simulink model "waterTankBurner"  (R2014b)
settings: Solver=ode1  StartTime=0.0  StopTime=100  FixedStep=0.0001  MaxStep=0.0001  RelTol=1e-3
(part 4 of 4)

== matlab function waterTankBurner/waterTank38/MATLAB Function1 ==
  data: x input; ode1 output; ode2 output; ode3 output; ode4 output
function [ode1,ode2,ode3,ode4] = ODEs(x)
%#codegen
K=0.075;
h=150;
ode1=0;
ode2=K*(h-x);
ode3=0;
ode4=-K*x;

== matlab function waterTankBurner/waterTank39/MATLAB Function ==
  data: q input; ON input; OFF input; x input; qNext output; reset output


function [qNext,reset]  = phi(q,  ON, OFF,x)
%#codegen


if q==1 % q=1, tank is in t1
    if ON==0
        qNext=1;
        reset=0;
    elseif ON==1
        qNext=2;
        reset=1;
    else
        qNext=-1;
        reset=-1;
    end;
    
elseif q==2 % q=2, tank is in t2
    if x<100 && OFF==0
        qNext=2;
        reset=0;
    elseif x>=100
        qNext=3;
        reset=1;
    elseif x<100 && OFF==1
        qNext=4;
        reset=1;
    else
        qNext=-1;
        reset=-1;
    end;

elseif q==3 % q=3, tank is in state t3
    if OFF==0
        qNext=3;
        reset=0;
    elseif OFF==1
        qNext=4;
        reset=1;
    else
        qNext=-1;
        reset=-1;
    end;
elseif q==4 % q=4, tank is in state t4
    if x>20 && ON==0
        qNext=4;
        reset=0;
    elseif x<=20
        qNext=1;
        reset=1;
    elseif x>20 && ON==1
        qNext=2;
        reset=1;
    else
        qNext=-1;
        reset=-1;
    end;
else
    qNext=-1; %this should never execute
    reset=-1;%this should never execute
end

== matlab function waterTankBurner/waterTank39/MATLAB Function1 ==
  data: x input; ode1 output; ode2 output; ode3 output; ode4 output
function [ode1,ode2,ode3,ode4] = ODEs(x)
%#codegen
K=0.075;
h=150;
ode1=0;
ode2=K*(h-x);
ode3=0;
ode4=-K*x;

== matlab function waterTankBurner/waterTank40/MATLAB Function ==
  data: q input; ON input; OFF input; x input; qNext output; reset output


function [qNext,reset]  = phi(q,  ON, OFF,x)
%#codegen


if q==1 % q=1, tank is in t1
    if ON==0
        qNext=1;
        reset=0;
    elseif ON==1
        qNext=2;
        reset=1;
    else
        qNext=-1;
        reset=-1;
    end;
    
elseif q==2 % q=2, tank is in t2
    if x<100 && OFF==0
        qNext=2;
        reset=0;
    elseif x>=100
        qNext=3;
        reset=1;
    elseif x<100 && OFF==1
        qNext=4;
        reset=1;
    else
        qNext=-1;
        reset=-1;
    end;

elseif q==3 % q=3, tank is in state t3
    if OFF==0
        qNext=3;
        reset=0;
    elseif OFF==1
        qNext=4;
        reset=1;
    else
        qNext=-1;
        reset=-1;
    end;
elseif q==4 % q=4, tank is in state t4
    if x>20 && ON==0
        qNext=4;
        reset=0;
    elseif x<=20
        qNext=1;
        reset=1;
    elseif x>20 && ON==1
        qNext=2;
        reset=1;
    else
        qNext=-1;
        reset=-1;
    end;
else
    qNext=-1; %this should never execute
    reset=-1;%this should never execute
end

== matlab function waterTankBurner/waterTank40/MATLAB Function1 ==
  data: x input; ode1 output; ode2 output; ode3 output; ode4 output
function [ode1,ode2,ode3,ode4] = ODEs(x)
%#codegen
K=0.075;
h=150;
ode1=0;
ode2=K*(h-x);
ode3=0;
ode4=-K*x;

== matlab function waterTankBurner/waterTank41/MATLAB Function ==
  data: q input; ON input; OFF input; x input; qNext output; reset output


function [qNext,reset]  = phi(q,  ON, OFF,x)
%#codegen


if q==1 % q=1, tank is in t1
    if ON==0
        qNext=1;
        reset=0;
    elseif ON==1
        qNext=2;
        reset=1;
    else
        qNext=-1;
        reset=-1;
    end;
    
elseif q==2 % q=2, tank is in t2
    if x<100 && OFF==0
        qNext=2;
        reset=0;
    elseif x>=100
        qNext=3;
        reset=1;
    elseif x<100 && OFF==1
        qNext=4;
        reset=1;
    else
        qNext=-1;
        reset=-1;
    end;

elseif q==3 % q=3, tank is in state t3
    if OFF==0
        qNext=3;
        reset=0;
    elseif OFF==1
        qNext=4;
        reset=1;
    else
        qNext=-1;
        reset=-1;
    end;
elseif q==4 % q=4, tank is in state t4
    if x>20 && ON==0
        qNext=4;
        reset=0;
    elseif x<=20
        qNext=1;
        reset=1;
    elseif x>20 && ON==1
        qNext=2;
        reset=1;
    else
        qNext=-1;
        reset=-1;
    end;
else
    qNext=-1; %this should never execute
    reset=-1;%this should never execute
end

== matlab function waterTankBurner/waterTank41/MATLAB Function1 ==
  data: x input; ode1 output; ode2 output; ode3 output; ode4 output
function [ode1,ode2,ode3,ode4] = ODEs(x)
%#codegen
K=0.075;
h=150;
ode1=0;
ode2=K*(h-x);
ode3=0;
ode4=-K*x;

== matlab function waterTankBurner/waterTank42/MATLAB Function ==
  data: q input; ON input; OFF input; x input; qNext output; reset output


function [qNext,reset]  = phi(q,  ON, OFF,x)
%#codegen


if q==1 % q=1, tank is in t1
    if ON==0
        qNext=1;
        reset=0;
    elseif ON==1
        qNext=2;
        reset=1;
    else
        qNext=-1;
        reset=-1;
    end;
    
elseif q==2 % q=2, tank is in t2
    if x<100 && OFF==0
        qNext=2;
        reset=0;
    elseif x>=100
        qNext=3;
        reset=1;
    elseif x<100 && OFF==1
        qNext=4;
        reset=1;
    else
        qNext=-1;
        reset=-1;
    end;

elseif q==3 % q=3, tank is in state t3
    if OFF==0
        qNext=3;
        reset=0;
    elseif OFF==1
        qNext=4;
        reset=1;
    else
        qNext=-1;
        reset=-1;
    end;
elseif q==4 % q=4, tank is in state t4
    if x>20 && ON==0
        qNext=4;
        reset=0;
    elseif x<=20
        qNext=1;
        reset=1;
    elseif x>20 && ON==1
        qNext=2;
        reset=1;
    else
        qNext=-1;
        reset=-1;
    end;
else
    qNext=-1; %this should never execute
    reset=-1;%this should never execute
end

== matlab function waterTankBurner/waterTank42/MATLAB Function1 ==
  data: x input; ode1 output; ode2 output; ode3 output; ode4 output
function [ode1,ode2,ode3,ode4] = ODEs(x)
%#codegen
K=0.075;
h=150;
ode1=0;
ode2=K*(h-x);
ode3=0;
ode4=-K*x;

== matlab function waterTankBurner/waterTank43/MATLAB Function ==
  data: q input; ON input; OFF input; x input; qNext output; reset output


function [qNext,reset]  = phi(q,  ON, OFF,x)
%#codegen


if q==1 % q=1, tank is in t1
    if ON==0
        qNext=1;
        reset=0;
    elseif ON==1
        qNext=2;
        reset=1;
    else
        qNext=-1;
        reset=-1;
    end;
    
elseif q==2 % q=2, tank is in t2
    if x<100 && OFF==0
        qNext=2;
        reset=0;
    elseif x>=100
        qNext=3;
        reset=1;
    elseif x<100 && OFF==1
        qNext=4;
        reset=1;
    else
        qNext=-1;
        reset=-1;
    end;

elseif q==3 % q=3, tank is in state t3
    if OFF==0
        qNext=3;
        reset=0;
    elseif OFF==1
        qNext=4;
        reset=1;
    else
        qNext=-1;
        reset=-1;
    end;
elseif q==4 % q=4, tank is in state t4
    if x>20 && ON==0
        qNext=4;
        reset=0;
    elseif x<=20
        qNext=1;
        reset=1;
    elseif x>20 && ON==1
        qNext=2;
        reset=1;
    else
        qNext=-1;
        reset=-1;
    end;
else
    qNext=-1; %this should never execute
    reset=-1;%this should never execute
end

== matlab function waterTankBurner/waterTank43/MATLAB Function1 ==
  data: x input; ode1 output; ode2 output; ode3 output; ode4 output
function [ode1,ode2,ode3,ode4] = ODEs(x)
%#codegen
K=0.075;
h=150;
ode1=0;
ode2=K*(h-x);
ode3=0;
ode4=-K*x;

== matlab function waterTankBurner/waterTank44/MATLAB Function ==
  data: q input; ON input; OFF input; x input; qNext output; reset output


function [qNext,reset]  = phi(q,  ON, OFF,x)
%#codegen


if q==1 % q=1, tank is in t1
    if ON==0
        qNext=1;
        reset=0;
    elseif ON==1
        qNext=2;
        reset=1;
    else
        qNext=-1;
        reset=-1;
    end;
    
elseif q==2 % q=2, tank is in t2
    if x<100 && OFF==0
        qNext=2;
        reset=0;
    elseif x>=100
        qNext=3;
        reset=1;
    elseif x<100 && OFF==1
        qNext=4;
        reset=1;
    else
        qNext=-1;
        reset=-1;
    end;

elseif q==3 % q=3, tank is in state t3
    if OFF==0
        qNext=3;
        reset=0;
    elseif OFF==1
        qNext=4;
        reset=1;
    else
        qNext=-1;
        reset=-1;
    end;
elseif q==4 % q=4, tank is in state t4
    if x>20 && ON==0
        qNext=4;
        reset=0;
    elseif x<=20
        qNext=1;
        reset=1;
    elseif x>20 && ON==1
        qNext=2;
        reset=1;
    else
        qNext=-1;
        reset=-1;
    end;
else
    qNext=-1; %this should never execute
    reset=-1;%this should never execute
end

== matlab function waterTankBurner/waterTank44/MATLAB Function1 ==
  data: x input; ode1 output; ode2 output; ode3 output; ode4 output
function [ode1,ode2,ode3,ode4] = ODEs(x)
%#codegen
K=0.075;
h=150;
ode1=0;
ode2=K*(h-x);
ode3=0;
ode4=-K*x;

== matlab function waterTankBurner/waterTank45/MATLAB Function ==
  data: q input; ON input; OFF input; x input; qNext output; reset output


function [qNext,reset]  = phi(q,  ON, OFF,x)
%#codegen


if q==1 % q=1, tank is in t1
    if ON==0
        qNext=1;
        reset=0;
    elseif ON==1
        qNext=2;
        reset=1;
    else
        qNext=-1;
        reset=-1;
    end;
    
elseif q==2 % q=2, tank is in t2
    if x<100 && OFF==0
        qNext=2;
        reset=0;
    elseif x>=100
        qNext=3;
        reset=1;
    elseif x<100 && OFF==1
        qNext=4;
        reset=1;
    else
        qNext=-1;
        reset=-1;
    end;

elseif q==3 % q=3, tank is in state t3
    if OFF==0
        qNext=3;
        reset=0;
    elseif OFF==1
        qNext=4;
        reset=1;
    else
        qNext=-1;
        reset=-1;
    end;
elseif q==4 % q=4, tank is in state t4
    if x>20 && ON==0
        qNext=4;
        reset=0;
    elseif x<=20
        qNext=1;
        reset=1;
    elseif x>20 && ON==1
        qNext=2;
        reset=1;
    else
        qNext=-1;
        reset=-1;
    end;
else
    qNext=-1; %this should never execute
    reset=-1;%this should never execute
end

== matlab function waterTankBurner/waterTank45/MATLAB Function1 ==
  data: x input; ode1 output; ode2 output; ode3 output; ode4 output
function [ode1,ode2,ode3,ode4] = ODEs(x)
%#codegen
K=0.075;
h=150;
ode1=0;
ode2=K*(h-x);
ode3=0;
ode4=-K*x;

== matlab function waterTankBurner/waterTank46/MATLAB Function ==
  data: q input; ON input; OFF input; x input; qNext output; reset output


function [qNext,reset]  = phi(q,  ON, OFF,x)
%#codegen


if q==1 % q=1, tank is in t1
    if ON==0
        qNext=1;
        reset=0;
    elseif ON==1
        qNext=2;
        reset=1;
    else
        qNext=-1;
        reset=-1;
    end;
    
elseif q==2 % q=2, tank is in t2
    if x<100 && OFF==0
        qNext=2;
        reset=0;
    elseif x>=100
        qNext=3;
        reset=1;
    elseif x<100 && OFF==1
        qNext=4;
        reset=1;
    else
        qNext=-1;
        reset=-1;
    end;

elseif q==3 % q=3, tank is in state t3
    if OFF==0
        qNext=3;
        reset=0;
    elseif OFF==1
        qNext=4;
        reset=1;
    else
        qNext=-1;
        reset=-1;
    end;
elseif q==4 % q=4, tank is in state t4
    if x>20 && ON==0
        qNext=4;
        reset=0;
    elseif x<=20
        qNext=1;
        reset=1;
    elseif x>20 && ON==1
        qNext=2;
        reset=1;
    else
        qNext=-1;
        reset=-1;
    end;
else
    qNext=-1; %this should never execute
    reset=-1;%this should never execute
end

== matlab function waterTankBurner/waterTank46/MATLAB Function1 ==
  data: x input; ode1 output; ode2 output; ode3 output; ode4 output
function [ode1,ode2,ode3,ode4] = ODEs(x)
%#codegen
K=0.075;
h=150;
ode1=0;
ode2=K*(h-x);
ode3=0;
ode4=-K*x;

== matlab function waterTankBurner/waterTank47/MATLAB Function ==
  data: q input; ON input; OFF input; x input; qNext output; reset output


function [qNext,reset]  = phi(q,  ON, OFF,x)
%#codegen


if q==1 % q=1, tank is in t1
    if ON==0
        qNext=1;
        reset=0;
    elseif ON==1
        qNext=2;
        reset=1;
    else
        qNext=-1;
        reset=-1;
    end;
    
elseif q==2 % q=2, tank is in t2
    if x<100 && OFF==0
        qNext=2;
        reset=0;
    elseif x>=100
        qNext=3;
        reset=1;
    elseif x<100 && OFF==1
        qNext=4;
        reset=1;
    else
        qNext=-1;
        reset=-1;
    end;

elseif q==3 % q=3, tank is in state t3
    if OFF==0
        qNext=3;
        reset=0;
    elseif OFF==1
        qNext=4;
        reset=1;
    else
        qNext=-1;
        reset=-1;
    end;
elseif q==4 % q=4, tank is in state t4
    if x>20 && ON==0
        qNext=4;
        reset=0;
    elseif x<=20
        qNext=1;
        reset=1;
    elseif x>20 && ON==1
        qNext=2;
        reset=1;
    else
        qNext=-1;
        reset=-1;
    end;
else
    qNext=-1; %this should never execute
    reset=-1;%this should never execute
end

== matlab function waterTankBurner/waterTank47/MATLAB Function1 ==
  data: x input; ode1 output; ode2 output; ode3 output; ode4 output
function [ode1,ode2,ode3,ode4] = ODEs(x)
%#codegen
K=0.075;
h=150;
ode1=0;
ode2=K*(h-x);
ode3=0;
ode4=-K*x;

== matlab function waterTankBurner/waterTank48/MATLAB Function ==
  data: q input; ON input; OFF input; x input; qNext output; reset output


function [qNext,reset]  = phi(q,  ON, OFF,x)
%#codegen


if q==1 % q=1, tank is in t1
    if ON==0
        qNext=1;
        reset=0;
    elseif ON==1
        qNext=2;
        reset=1;
    else
        qNext=-1;
        reset=-1;
    end;
    
elseif q==2 % q=2, tank is in t2
    if x<100 && OFF==0
        qNext=2;
        reset=0;
    elseif x>=100
        qNext=3;
        reset=1;
    elseif x<100 && OFF==1
        qNext=4;
        reset=1;
    else
        qNext=-1;
        reset=-1;
    end;

elseif q==3 % q=3, tank is in state t3
    if OFF==0
        qNext=3;
        reset=0;
    elseif OFF==1
        qNext=4;
        reset=1;
    else
        qNext=-1;
        reset=-1;
    end;
elseif q==4 % q=4, tank is in state t4
    if x>20 && ON==0
        qNext=4;
        reset=0;
    elseif x<=20
        qNext=1;
        reset=1;
    elseif x>20 && ON==1
        qNext=2;
        reset=1;
    else
        qNext=-1;
        reset=-1;
    end;
else
    qNext=-1; %this should never execute
    reset=-1;%this should never execute
end

== matlab function waterTankBurner/waterTank48/MATLAB Function1 ==
  data: x input; ode1 output; ode2 output; ode3 output; ode4 output
function [ode1,ode2,ode3,ode4] = ODEs(x)
%#codegen
K=0.075;
h=150;
ode1=0;
ode2=K*(h-x);
ode3=0;
ode4=-K*x;

== matlab function waterTankBurner/waterTank49/MATLAB Function ==
  data: q input; ON input; OFF input; x input; qNext output; reset output


function [qNext,reset]  = phi(q,  ON, OFF,x)
%#codegen


if q==1 % q=1, tank is in t1
    if ON==0
        qNext=1;
        reset=0;
    elseif ON==1
        qNext=2;
        reset=1;
    else
        qNext=-1;
        reset=-1;
    end;
    
elseif q==2 % q=2, tank is in t2
    if x<100 && OFF==0
        qNext=2;
        reset=0;
    elseif x>=100
        qNext=3;
        reset=1;
    elseif x<100 && OFF==1
        qNext=4;
        reset=1;
    else
        qNext=-1;
        reset=-1;
    end;

elseif q==3 % q=3, tank is in state t3
    if OFF==0
        qNext=3;
        reset=0;
    elseif OFF==1
        qNext=4;
        reset=1;
    else
        qNext=-1;
        reset=-1;
    end;
elseif q==4 % q=4, tank is in state t4
    if x>20 && ON==0
        qNext=4;
        reset=0;
    elseif x<=20
        qNext=1;
        reset=1;
    elseif x>20 && ON==1
        qNext=2;
        reset=1;
    else
        qNext=-1;
        reset=-1;
    end;
else
    qNext=-1; %this should never execute
    reset=-1;%this should never execute
end

== matlab function waterTankBurner/waterTank49/MATLAB Function1 ==
  data: x input; ode1 output; ode2 output; ode3 output; ode4 output
function [ode1,ode2,ode3,ode4] = ODEs(x)
%#codegen
K=0.075;
h=150;
ode1=0;
ode2=K*(h-x);
ode3=0;
ode4=-K*x;
